simulink model "MultiSensorsR2014a"  (R2016b)
settings: Solver=ode45  StartTime=0.0  StopTime=5  MaxStep=0.01  RelTol=1e-3  EnableMultiTasking=on
InitFcn:
  | WhiteNoise_Mean=0;
  | WhiteNoise_Variance=1;
  | 
  | WhiteNoise_Mean2=0;
  | WhiteNoise_Variance2=1;
  | 
  | F_amplitude = 1;
  | F_frequency =10; % rad/s
  | 
  | beta=1000;
  | 
  | dt = 0.01;
libraries: commnoisgen2 x2
settings Model: Creator=suki  LastModifiedBy=DMori
settings DataIOCC: LimitDataPoints=on  SaveFormat=Array
settings OptimizationCC: LifeSpan=inf
settings DebuggingCC: SolverPrmCheckMsg=warning  SFUnexpectedBacktrackingDiag=warning  SFNoUnconditionalDefaultTransitionDiag=warning  SFExecutionAtInitializationDiag=none
settings HardwareCC: ProdBitPerPointer=32  ProdBitPerSizeT=32  ProdBitPerPtrDiffT=32  ProdLargestAtomicFloat=None  ProdIntDivRoundTo=Undefined  ProdEndianess=Unspecified  ProdWordSize=32  ProdHWDeviceType=32-bit Generic
settings ModelReferenceCC: PropagateSignalLabelsOutOfModel=off
settings GRTTargetCC: TargetLangStandard=C89/C90 (ANSI)  GeneratePreprocessorConditionals=Disable all
settings ConfigComp: CovMetricSettings=dw  CovHtmlReporting=on  CovSaveCumulativeToWorkspaceVar=on  CovSaveSingleToWorkspaceVar=on  CovExternalEMLEnable=off  CovSFcnEnable=off

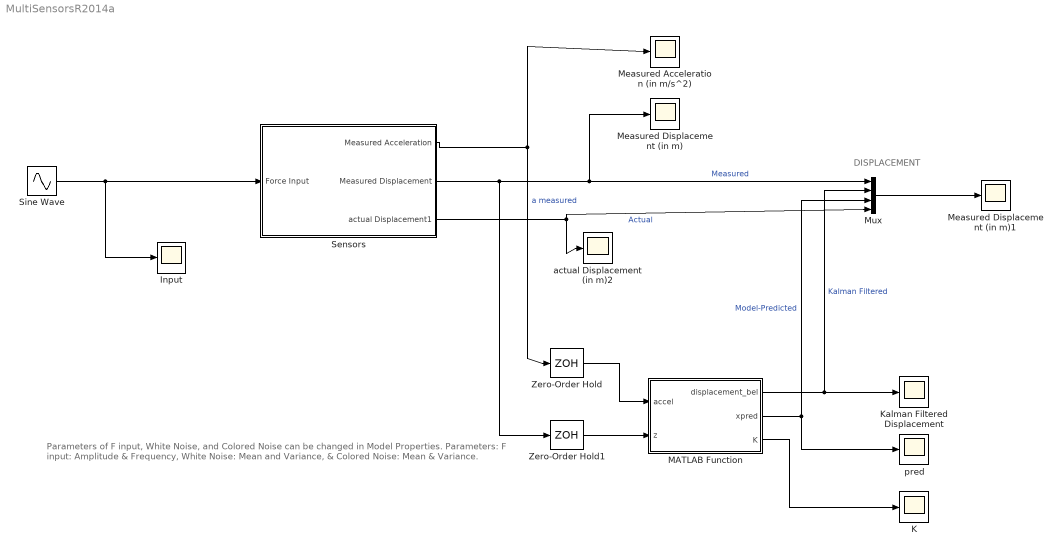
== system MultiSensorsR2014a ==
  note: DISPLACEMENT
  note: Parameters of F input, White Noise, and Colored Noise can be changed in Model Properties.
      |
      | Parameters:
      | F input: Amplitude & Frequency,
      | White Noise: Mean and Variance, &
      | Colored Noise: Mean & Variance.
  Input : Scope
  K : Scope
  Kalman Filtered Displacement : Scope
  MATLAB Function : MATLAB Function  TreatAsAtomicUnit=on
  Measured Acceleration (in m/s^2) : Scope
  Measured Displacement (in m) : Scope
  Measured Displacement (in m)1 : Scope
  Mux : Mux
  Sensors : Subsystem
  Sine Wave : Sin  Amplitude=F_amplitude  Frequency=F_frequency  Phase=6*rand  SampleTime=0
  Zero-Order Hold : ZeroOrderHold  SampleTime=dt
  Zero-Order Hold1 : ZeroOrderHold  SampleTime=dt
  actual Displacement (in m)2 : Scope
  pred : Scope
  wires:
  Sensors/1(Measured Acceleration) -> Zero-Order Hold/1, Measured Acceleration (in m/s^2)/1  "a measured"
  Sensors/2(Measured Displacement) -> Zero-Order Hold1/1, Mux/1, Measured Displacement (in m)/1  "Measured"
  Sine Wave/1 -> Input/1, Sensors/1(Force Input)
  MATLAB Function/1(displacement_bel) -> Mux/2, Kalman Filtered Displacement/1  "Kalman Filtered"
  MATLAB Function/2(xpred) -> pred/1, Mux/3  "Model-Predicted"
  Mux/1 -> Measured Displacement (in m)1/1
  Sensors/3(actual Displacement1) -> actual Displacement (in m)2/1, Mux/4  "Actual"
  Zero-Order Hold/1 -> MATLAB Function/1(accel)
  Zero-Order Hold1/1 -> MATLAB Function/2(z)
  MATLAB Function/3(K) -> K/1

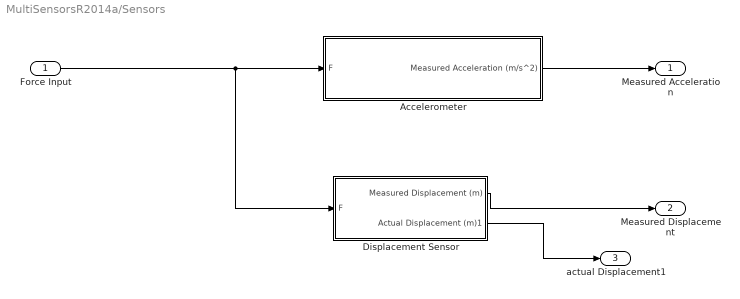
== system MultiSensorsR2014a/Sensors ==
  Force Input : Inport
  Accelerometer : Subsystem
  Displacement Sensor : Subsystem
  Measured Acceleration : Outport
  Measured Displacement : Outport  Port=2
  actual Displacement1 : Outport  Port=3
  wires:
  Force Input/1 -> Accelerometer/1(F), Displacement Sensor/1(F)
  Displacement Sensor/1(Measured Displacement (m)) -> Measured Displacement/1
  Accelerometer/1(Measured Acceleration (m/s^2)) -> Measured Acceleration/1
  Displacement Sensor/2(Actual Displacement (m)1) -> actual Displacement1/1

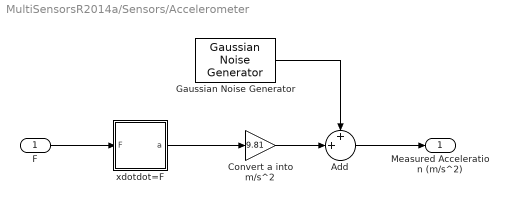
== system MultiSensorsR2014a/Sensors/Accelerometer ==
  F : Inport
  Add : Sum  Inputs=++|
  Convert a into m/s^2 : Gain  Gain=9.81
  Gaussian Noise Generator : commnoisgen2/Gaussian Noise Generator  m=WhiteNoise_Mean  d=WhiteNoise_Variance  s=41  Ts=0.01  frameBased=off  sampPerFrame=1  orient=off  outDataType=double
  xdotdot=F : Subsystem
  Measured Acceleration (m/s^2) : Outport
  wires:
  F/1 -> xdotdot=F/1(F)
  Gaussian Noise Generator/1 -> Add/1
  Convert a into m/s^2/1 -> Add/2
  xdotdot=F/1(a) -> Convert a into m/s^2/1
  Add/1 -> Measured Acceleration (m/s^2)/1

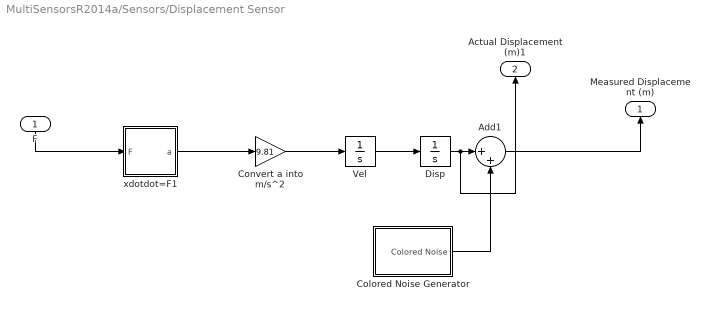
== system MultiSensorsR2014a/Sensors/Displacement Sensor ==
  F : Inport
  Add1 : Sum  Inputs=|++
  Colored Noise Generator : Subsystem
  Convert a into m/s^2 : Gain  Gain=9.81
  Disp : Integrator
  Vel : Integrator
  xdotdot=F1 : Subsystem
  Measured Displacement (m) : Outport
  Actual Displacement (m)1 : Outport  Port=2
  wires:
  Colored Noise Generator/1(Colored Noise) -> Add1/2
  F/1 -> xdotdot=F1/1(F)
  Add1/1 -> Measured Displacement (m)/1
  Disp/1 -> Actual Displacement (m)1/1, Add1/1
  Vel/1 -> Disp/1
  xdotdot=F1/1(a) -> Convert a into m/s^2/1
  Convert a into m/s^2/1 -> Vel/1

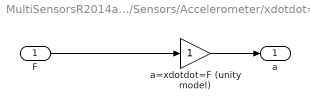
== system MultiSensorsR2014a/Sensors/Accelerometer/xdotdot=F ==
  F : Inport
  a=xdotdot=F (unity model) : Gain
  a : Outport
  wires:
  F/1 -> a=xdotdot=F (unity model)/1
  a=xdotdot=F (unity model)/1 -> a/1

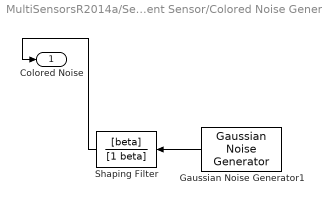
== system MultiSensorsR2014a/Sensors/Displacement Sensor/Colored Noise Generator ==
  Gaussian Noise Generator1 : commnoisgen2/Gaussian Noise Generator  m=WhiteNoise_Mean2  d=WhiteNoise_Variance2  s=20  Ts=0.01  frameBased=off  sampPerFrame=1  orient=off  outDataType=double
  Shaping Filter : TransferFcn  Numerator=[beta]  Denominator=[1 beta]
  Colored Noise : Outport
  wires:
  Shaping Filter/1 -> Colored Noise/1
  Gaussian Noise Generator1/1 -> Shaping Filter/1

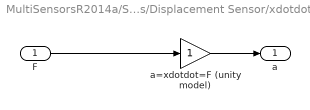
== system MultiSensorsR2014a/Sensors/Displacement Sensor/xdotdot=F1 ==
  F : Inport
  a=xdotdot=F (unity model) : Gain
  a : Outport
  wires:
  F/1 -> a=xdotdot=F (unity model)/1
  a=xdotdot=F (unity model)/1 -> a/1

== matlab function MultiSensorsR2014a/MATLAB Function ==
  data: accel input; z input; displacement_bel output; xpred output; K output
function [displacement_bel, xpred, K] = KF(accel,z)
persistent xbel
persistent Pbel
persistent xmodel

if isempty(xbel)
    xbel = [0; 0];
end
if isempty(Pbel)
    Pbel = [1 0; 0 1];
end
if isempty(xmodel)
    xmodel = [0; 0];
end

%%%%%Kalman Filter Parameters
dt = 0.01;
%continuous SS
% A = [0 1; 0 0];
% B = [0; 1];
% C = [1 0];
% D = 0;
%Discrete SS
A = [0 1; -1 2];
B = [0; dt^2];
C = [1 0];
D = 0;

Q=[1 0; 0 1];
R = 100*dt^4;

%model only
xmodel = A*xmodel + B*accel;

%kalman filtered
x = A*xbel + B*accel;
P = A*Pbel*A' + Q;

% xbel = x;
K = P*C'*inv(C*P*C'+R);
%   K=[1.618; 1];
xbel = x-K*(C*x-z);
Pbel=(eye(2)-K*C)*P;

xpred = xmodel(1);
displacement_bel = C*xbel;
